simulink model "KillerWhaleModel"  (R2020b)
settings: Solver=ode15s  StartTime=0.0  StopTime=10.0  MaxStep=0.01  RelTol=1e-3
model workspace: external: MATLAB File KillerWhaleParams.m (data not in the file)
undefined symbols (not defined in the file or in its folder): frontParams, rearParams, standParams, X, Y, Z
libraries: sm_lib x4076, nesl_utility x6
(part 2 of 62)

== system KillerWhaleModel/WhaleStand ==
  J5 : Inport
  PitchLink1_1 : Subsystem
      settings: PortSchema="{\"entries\":[{\"content\":{\"sides\":[{\"content\":{\"connectorIds\":[\"LConn1\"]},\"type\":\"ConnectorPlacement.EquallySpacedRectSide\",\"uuid\":\"daed8036-1c83-499a-be75-c3d6daf1be0e\"},{\"content\":{\"connectorIds\":[\"RConn1\"],\"side\":\"RIGHT\"},\"type\":\"ConnectorPlacement.EquallySpacedRectSide\",\"uuid\":\"d51b8bb5-d322-4cdc-bb54-b3adc448b83e\"},{\"content\":{\"connectorIds\":[],\"side\":\"TOP\"},\"type\":\"ConnectorPlacement.EquallySpacedRectSide\",\"uuid\":\"6033db49-1de1-4080-b1d2-f43e71cbe144\"},{\"content\":{\"connectorIds\":[\"RConn2\",\"RConn3\"],\"side\":\"BOTTOM\"},\"type\":\"ConnectorPlacement.EquallySpacedRectSide\",\"uuid\":\"5e0a4000-b8ff-4240-85b3-c85b6cef6958\"},{\"content\":{\"connectorIds\":[],\"side\":\"HIDDEN\"},\"type\":\"ConnectorPlacement.EquallySpacedRectSide\",\"uuid\":\"849e2ead-7697-44fd-a88a-81f8afad95b9\"}]},\"type\":\"ConnectorPlacement.EquallySpacedConnector\",\"uuid\":\"26ddce31-1319-410d-869c-816121a0afb6\"}],\"packageUris\":[\"http://schema.mathworks.com/mf0/Connector/R2020b\"],\"version\":\"1.0\"}"
  PitchLink2_1 : Subsystem
  PitchLink3_1 : Subsystem
      settings: PortSchema="{\"entries\":[{\"content\":{\"sides\":[{\"content\":{\"connectorIds\":[\"LConn1\"]},\"type\":\"ConnectorPlacement.EquallySpacedRectSide\",\"uuid\":\"ffe909db-c886-4e63-ba46-0b3ec8f48d0a\"},{\"content\":{\"connectorIds\":[\"RConn1\"],\"side\":\"RIGHT\"},\"type\":\"ConnectorPlacement.EquallySpacedRectSide\",\"uuid\":\"77d7e64e-07ff-4cea-8643-07133e8c2799\"},{\"content\":{\"connectorIds\":[\"LConn2\"],\"side\":\"TOP\"},\"type\":\"ConnectorPlacement.EquallySpacedRectSide\",\"uuid\":\"189798a8-90a9-455e-91d8-3d815b26c78b\"},{\"content\":{\"connectorIds\":[\"RConn2\"],\"side\":\"BOTTOM\"},\"type\":\"ConnectorPlacement.EquallySpacedRectSide\",\"uuid\":\"6ca3684c-b3f7-48ad-a60e-7715eeec248c\"},{\"content\":{\"connectorIds\":[],\"side\":\"HIDDEN\"},\"type\":\"ConnectorPlacement.EquallySpacedRectSide\",\"uuid\":\"9488b140-3c37-4540-8da6-f5b0cd01be8e\"}]},\"type\":\"ConnectorPlacement.EquallySpacedConnector\",\"uuid\":\"c943227e-23c5-4cc6-8f81-35f98998dc73\"}],\"packageUris\":[\"http://schema.mathworks.com/mf0/Connector/R2020b\"],\"version\":\"1.0\"}"
  PitchLink4_1 : Subsystem
  Revolute1 : sm_lib/Joints/Revolute Joint  JointMode=Normal  SenseConstraintForce=off  SenseConstraintForceX=off  SenseConstraintForceY=off  SenseConstraintForceZ=off  SenseConstraintTorque=off  SenseConstraintTorqueX=off  SenseConstraintTorqueY=off  SenseConstraintTorqueZ=off  SenseTotalForce=off  SenseTotalForceX=off  SenseTotalForceY=off  SenseTotalForceZ=off  SenseTotalTorque=off  SenseTotalTorqueX=off  SenseTotalTorqueY=off  SenseTotalTorqueZ=off  CompositeWrenchDir=FollowerOnBase  CompositeWrenchFrame=BaseFrame  EquilibriumPosition=0  EquilibriumPositionUnits=deg  SpringStiffness=0  SpringStiffnessUnits=N*m/deg  DampingCoefficient=0  DampingCoefficientUnits=N*m/(deg/s)  TorqueActuationMode=NoTorque  MotionActuationMode=ComputedMotion  SensePosition=off  SenseVelocity=off  SenseAcceleration=off  SenseTorqueForce=off  SenseLowerLimitTorqueForce=off  SenseUpperLimitTorqueForce=off  LowerLimitSpecify=off  LowerLimitBound=-90  LowerLimitBoundUnits=deg  LowerLimitStiffness=1e4  LowerLimitStiffnessUnits=N*m/deg  LowerLimitDamping=10  LowerLimitDampingUnits=N*m/(deg/s)  LowerLimitTransitionRegionWidth=0.1  LowerLimitTransitionRegionWidthUnits=deg  UpperLimitSpecify=off  UpperLimitBound=90  UpperLimitBoundUnits=deg  UpperLimitStiffness=1e4  UpperLimitStiffnessUnits=N*m/deg  UpperLimitDamping=10  UpperLimitDampingUnits=N*m/(deg/s)  UpperLimitTransitionRegionWidth=0.1  UpperLimitTransitionRegionWidthUnits=deg  PositionTargetSpecify=off  PositionTargetPriority=Low  PositionTargetValue=standParams.RevoluteJoint(1).Rz.Pos  PositionTargetValueUnits=deg  VelocityTargetSpecify=off  VelocityTargetPriority=High  VelocityTargetValue=0  VelocityTargetValueUnits=deg/s
  Revolute2 : sm_lib/Joints/Revolute Joint  JointMode=Normal  SenseConstraintForce=off  SenseConstraintForceX=off  SenseConstraintForceY=off  SenseConstraintForceZ=off  SenseConstraintTorque=off  SenseConstraintTorqueX=off  SenseConstraintTorqueY=off  SenseConstraintTorqueZ=off  SenseTotalForce=off  SenseTotalForceX=off  SenseTotalForceY=off  SenseTotalForceZ=off  SenseTotalTorque=off  SenseTotalTorqueX=off  SenseTotalTorqueY=off  SenseTotalTorqueZ=off  CompositeWrenchDir=FollowerOnBase  CompositeWrenchFrame=BaseFrame  EquilibriumPosition=0  EquilibriumPositionUnits=deg  SpringStiffness=0  SpringStiffnessUnits=N*m/deg  DampingCoefficient=0  DampingCoefficientUnits=N*m/(deg/s)  TorqueActuationMode=NoTorque  MotionActuationMode=ComputedMotion  SensePosition=off  SenseVelocity=off  SenseAcceleration=off  SenseTorqueForce=off  SenseLowerLimitTorqueForce=off  SenseUpperLimitTorqueForce=off  LowerLimitSpecify=off  LowerLimitBound=-90  LowerLimitBoundUnits=deg  LowerLimitStiffness=1e4  LowerLimitStiffnessUnits=N*m/deg  LowerLimitDamping=10  LowerLimitDampingUnits=N*m/(deg/s)  LowerLimitTransitionRegionWidth=0.1  LowerLimitTransitionRegionWidthUnits=deg  UpperLimitSpecify=off  UpperLimitBound=90  UpperLimitBoundUnits=deg  UpperLimitStiffness=1e4  UpperLimitStiffnessUnits=N*m/deg  UpperLimitDamping=10  UpperLimitDampingUnits=N*m/(deg/s)  UpperLimitTransitionRegionWidth=0.1  UpperLimitTransitionRegionWidthUnits=deg  PositionTargetSpecify=off  PositionTargetPriority=High  PositionTargetValue=0  PositionTargetValueUnits=deg  VelocityTargetSpecify=off  VelocityTargetPriority=High  VelocityTargetValue=0  VelocityTargetValueUnits=deg/s
  Revolute3 : sm_lib/Joints/Revolute Joint  JointMode=Normal  SenseConstraintForce=off  SenseConstraintForceX=off  SenseConstraintForceY=off  SenseConstraintForceZ=off  SenseConstraintTorque=off  SenseConstraintTorqueX=off  SenseConstraintTorqueY=off  SenseConstraintTorqueZ=off  SenseTotalForce=off  SenseTotalForceX=off  SenseTotalForceY=off  SenseTotalForceZ=off  SenseTotalTorque=off  SenseTotalTorqueX=off  SenseTotalTorqueY=off  SenseTotalTorqueZ=off  CompositeWrenchDir=FollowerOnBase  CompositeWrenchFrame=BaseFrame  EquilibriumPosition=0  EquilibriumPositionUnits=deg  SpringStiffness=0  SpringStiffnessUnits=N*m/deg  DampingCoefficient=0  DampingCoefficientUnits=N*m/(deg/s)  TorqueActuationMode=NoTorque  MotionActuationMode=ComputedMotion  SensePosition=off  SenseVelocity=off  SenseAcceleration=off  SenseTorqueForce=off  SenseLowerLimitTorqueForce=off  SenseUpperLimitTorqueForce=off  LowerLimitSpecify=off  LowerLimitBound=-90  LowerLimitBoundUnits=deg  LowerLimitStiffness=1e4  LowerLimitStiffnessUnits=N*m/deg  LowerLimitDamping=10  LowerLimitDampingUnits=N*m/(deg/s)  LowerLimitTransitionRegionWidth=0.1  LowerLimitTransitionRegionWidthUnits=deg  UpperLimitSpecify=off  UpperLimitBound=90  UpperLimitBoundUnits=deg  UpperLimitStiffness=1e4  UpperLimitStiffnessUnits=N*m/deg  UpperLimitDamping=10  UpperLimitDampingUnits=N*m/(deg/s)  UpperLimitTransitionRegionWidth=0.1  UpperLimitTransitionRegionWidthUnits=deg  PositionTargetSpecify=on  PositionTargetPriority=Low  PositionTargetValue=standParams.RevoluteJoint(3).Rz.Pos  PositionTargetValueUnits=deg  VelocityTargetSpecify=off  VelocityTargetPriority=High  VelocityTargetValue=0  VelocityTargetValueUnits=deg/s
  Revolute4 : sm_lib/Joints/Revolute Joint  JointMode=Normal  SenseConstraintForce=off  SenseConstraintForceX=off  SenseConstraintForceY=off  SenseConstraintForceZ=off  SenseConstraintTorque=off  SenseConstraintTorqueX=off  SenseConstraintTorqueY=off  SenseConstraintTorqueZ=off  SenseTotalForce=off  SenseTotalForceX=off  SenseTotalForceY=off  SenseTotalForceZ=off  SenseTotalTorque=off  SenseTotalTorqueX=off  SenseTotalTorqueY=off  SenseTotalTorqueZ=off  CompositeWrenchDir=FollowerOnBase  CompositeWrenchFrame=BaseFrame  EquilibriumPosition=0  EquilibriumPositionUnits=deg  SpringStiffness=0  SpringStiffnessUnits=N*m/deg  DampingCoefficient=0  DampingCoefficientUnits=N*m/(deg/s)  TorqueActuationMode=ComputedTorque  MotionActuationMode=InputMotion  SensePosition=off  SenseVelocity=off  SenseAcceleration=off  SenseTorqueForce=off  SenseLowerLimitTorqueForce=off  SenseUpperLimitTorqueForce=off  LowerLimitSpecify=on  LowerLimitBound=-12.5  LowerLimitBoundUnits=deg  LowerLimitStiffness=1e4  LowerLimitStiffnessUnits=N*m/deg  LowerLimitDamping=1e3  LowerLimitDampingUnits=N*m/(deg/s)  LowerLimitTransitionRegionWidth=0.5  LowerLimitTransitionRegionWidthUnits=deg  UpperLimitSpecify=on  UpperLimitBound=41.5  UpperLimitBoundUnits=deg  UpperLimitStiffness=1e4  UpperLimitStiffnessUnits=N*m/deg  UpperLimitDamping=1e3  UpperLimitDampingUnits=N*m/(deg/s)  UpperLimitTransitionRegionWidth=0.5  UpperLimitTransitionRegionWidthUnits=deg  PositionTargetSpecify=on  PositionTargetPriority=Low  PositionTargetValue=standParams.RevoluteJoint(2).Rz.Pos  PositionTargetValueUnits=deg  VelocityTargetSpecify=off  VelocityTargetPriority=High  VelocityTargetValue=0  VelocityTargetValueUnits=deg/s
  Simulink-PS Converter : nesl_utility/Simulink-PS Converter  PhysicalDomain=network_engine_domain  SubClassName=ps_input  LeftPortType=input  RightPortType=output  PseudoPeriodic=off  Frequencies=[]  NoiseDistribution=none  NoiseParameters=[]  Unit=deg  AffineConversion=off  FilteringAndDerivatives=filter  SimscapeFilterOrder=2  InputFilterTimeConstant=0.01  UdotUserProvided=0
  S1 : PMIOPort  Side=Left
  S2 : PMIOPort  Port=2  Side=Left
  wires:
  J5/1 -> Simulink-PS Converter/1
  connections:
  PitchLink3_1/LConn1 -- Revolute3/RConn1
  PitchLink1_1/LConn1 -- Revolute2/RConn1
  PitchLink2_1/RConn2 -- Revolute3/LConn1
  PitchLink4_1/LConn1 -- Revolute4/RConn1
  PitchLink2_1/RConn1 -- Revolute2/LConn1
  PitchLink4_1/LConn2 -- Revolute1/RConn1
  PitchLink1_1/RConn1 -- Revolute4/LConn1
  PitchLink3_1/RConn1 -- Revolute1/LConn1
  S1/RConn1 -- PitchLink3_1/RConn2
  PitchLink4_1/RConn1 -- S2/RConn1
  Simulink-PS Converter/RConn1 -- Revolute4/LConn2

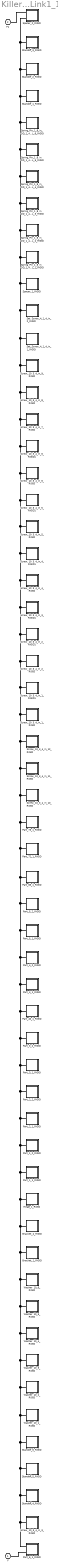
== system KillerWhaleModel/HeadLinkage/HeadLink1_1 ==
  Bracket_1_RIGID : Subsystem
  Bracket_2_RIGID : Subsystem
  Hinge_1_RIGID : Subsystem
  Part_1_1_RIGID : Subsystem
  Part_1_2_RIGID : Subsystem
  Part_2_1_RIGID : Subsystem
  Part_2_2_RIGID : Subsystem
  Part_3_1_RIGID : Subsystem
  Part_3_2_RIGID : Subsystem
  Part_40_1_RIGID : Subsystem
  Part_4_1_RIGID : Subsystem
  Part_4_2_RIGID : Subsystem
  Part_5_1_RIGID : Subsystem
  Part_5_2_RIGID : Subsystem
  Part_65_1_RIGID : Subsystem
  Part_6_1_RIGID : Subsystem
  Part_72_1_RIGID : Subsystem
  Part_73_1_RIGID : Subsystem
  Screw_10_3_4_in_10_RIGID : Subsystem
  Screw_10_3_4_in_11_RIGID : Subsystem
  Screw_10_3_4_in_12_RIGID : Subsystem
  Screw_10_3_4_in_1_RIGID : Subsystem
  Screw_10_3_4_in_1_RIGID1 : Subsystem
  Screw_10_3_4_in_2_RIGID : Subsystem
  Screw_10_3_4_in_2_RIGID1 : Subsystem
  Screw_10_3_4_in_3_RIGID : Subsystem
  Screw_10_3_4_in_3_RIGID1 : Subsystem
  Screw_10_3_4_in_4_RIGID : Subsystem
  Screw_10_3_4_in_4_RIGID1 : Subsystem
  Screw_10_3_4_in_5_RIGID : Subsystem
  Screw_10_3_4_in_5_RIGID1 : Subsystem
  Screw_10_3_4_in_6_RIGID : Subsystem
  Screw_10_3_4_in_6_RIGID1 : Subsystem
  Screw_10_3_4_in_7_RIGID : Subsystem
  Screw_10_3_4_in_8_RIGID : Subsystem
  Screw_10_3_4_in_9_RIGID : Subsystem
  Set_Screw_4_1_4_in_1_RIGID : Subsystem
  Set_Screw_4_1_4_in_2_RIGID : Subsystem
  Spacer_1_RIGID : Subsystem
  Spacer_2_RIGID : Subsystem
  Spring_Pin_1_8_in_OD_1_4_in_L_1_RIGID : Subsystem
  Spring_Pin_1_8_in_OD_1_4_in_L_2_RIGID : Subsystem
  Spring_Pin_1_8_in_OD_1_4_in_L_3_RIGID : Subsystem
  Spring_Pin_1_8_in_OD_1_4_in_L_4_RIGID : Subsystem
  Spring_Pin_1_8_in_OD_1_4_in_L_5_RIGID : Subsystem
  Spring_Pin_1_8_in_OD_1_4_in_L_6_RIGID : Subsystem
  Standoff_1_RIGID : Subsystem
  Standoff_2_RIGID : Subsystem
  Standoff_3_RIGID : Subsystem
  Standoff_4_RIGID : Subsystem
  Standoff_5_RIGID : Subsystem
  Standoff_6_RIGID : Subsystem
  Washer_10_1_RIGID : Subsystem
  Washer_10_2_RIGID : Subsystem
  Washer_10_3_RIGID : Subsystem
  Washer_10_4_RIGID : Subsystem
  Washer_10_5_RIGID : Subsystem
  Washer_10_6_RIGID : Subsystem
  F : PMIOPort  Side=Left
  F1 : PMIOPort  Port=2  Side=Right
  connections:
  Bracket_1_RIGID/LConn1 -- Part_6_1_RIGID/LConn1 -- Screw_10_3_4_in_3_RIGID/LConn1 -- Standoff_4_RIGID/LConn1 -- Standoff_5_RIGID/LConn1 -- Standoff_6_RIGID/LConn1 -- Washer_10_1_RIGID/LConn1 -- Washer_10_2_RIGID/LConn1 -- Washer_10_3_RIGID/LConn1 -- Washer_10_4_RIGID/LConn1 -- Washer_10_5_RIGID/LConn1 -- Washer_10_6_RIGID/LConn1 -- Spacer_2_RIGID/LConn2 -- Standoff_3_RIGID/LConn1 -- Standoff_2_RIGID/LConn1 -- Standoff_1_RIGID/LConn1 -- Spring_Pin_1_8_in_OD_1_4_in_L_6_RIGID/LConn1 -- Spring_Pin_1_8_in_OD_1_4_in_L_5_RIGID/LConn1 -- Spring_Pin_1_8_in_OD_1_4_in_L_4_RIGID/LConn1 -- Spring_Pin_1_8_in_OD_1_4_in_L_3_RIGID/LConn1 -- Spring_Pin_1_8_in_OD_1_4_in_L_2_RIGID/LConn1 -- Spring_Pin_1_8_in_OD_1_4_in_L_1_RIGID/LConn1 -- Spacer_1_RIGID/LConn1 -- Set_Screw_4_1_4_in_2_RIGID/LConn1 -- Set_Screw_4_1_4_in_1_RIGID/LConn1 -- Screw_10_3_4_in_9_RIGID/LConn1 -- Screw_10_3_4_in_8_RIGID/LConn1 -- Screw_10_3_4_in_7_RIGID/LConn1 -- Screw_10_3_4_in_6_RIGID1/LConn1 -- Screw_10_3_4_in_6_RIGID/LConn1 -- Screw_10_3_4_in_5_RIGID1/LConn1 -- Screw_10_3_4_in_5_RIGID/LConn1 -- Screw_10_3_4_in_4_RIGID1/LConn1 -- Screw_10_3_4_in_4_RIGID/LConn1 -- Screw_10_3_4_in_3_RIGID1/LConn1 -- Screw_10_3_4_in_2_RIGID1/LConn1 -- Screw_10_3_4_in_2_RIGID/LConn1 -- Screw_10_3_4_in_1_RIGID1/LConn1 -- Screw_10_3_4_in_1_RIGID/LConn1 -- Screw_10_3_4_in_12_RIGID/LConn1 -- Screw_10_3_4_in_11_RIGID/LConn1 -- Screw_10_3_4_in_10_RIGID/LConn1 -- Part_73_1_RIGID/LConn1 -- Part_72_1_RIGID/LConn1 -- Part_65_1_RIGID/LConn1 -- Part_5_2_RIGID/LConn1 -- Part_5_1_RIGID/LConn1 -- Part_4_2_RIGID/LConn1 -- Part_4_1_RIGID/LConn1 -- Part_40_1_RIGID/LConn1 -- Part_3_2_RIGID/LConn1 -- Part_3_1_RIGID/LConn1 -- Part_2_2_RIGID/LConn1 -- Part_2_1_RIGID/LConn1 -- Part_1_2_RIGID/LConn1 -- Part_1_1_RIGID/LConn1 -- Hinge_1_RIGID/LConn1 -- Bracket_2_RIGID/LConn1
  Part_6_1_RIGID/LConn2 -- F/RConn1
  Spacer_2_RIGID/LConn1 -- F1/RConn1

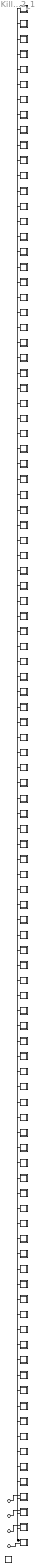
== system KillerWhaleModel/HeadLinkage/HeadLink2_1 ==
  Frame_Part_1_RIGID : Subsystem
  Frame_Part_2_RIGID : Subsystem
  Part_1_1_RIGID : Subsystem
  Part_1_2_RIGID : Subsystem
  Part_1_3_RIGID : Subsystem
  Part_1_4_RIGID : Subsystem
  Part_24_1_RIGID : Subsystem
  Part_24r_1_RIGID : Subsystem
  Part_2_1_RIGID : Subsystem
  Part_2_2_RIGID : Subsystem
  Part_2_3_RIGID : Subsystem
  Part_2_4_RIGID : Subsystem
  Part_3_1_RIGID : Subsystem
  Part_3_2_RIGID : Subsystem
  Part_3_3_RIGID : Subsystem
  Part_3_4_RIGID : Subsystem
  Part_4_1_RIGID : Subsystem
  Part_4_2_RIGID : Subsystem
  Part_4_3_RIGID : Subsystem
  Part_4_4_RIGID : Subsystem
  Part_5_1_RIGID : Subsystem
  Part_5_2_RIGID : Subsystem
  Part_5_3_RIGID : Subsystem
  Part_5_4_RIGID : Subsystem
  Part_6_1_RIGID : Subsystem
  Part_6_2_RIGID : Subsystem
  Part_809_1_RIGID : Subsystem
  Part_809_2_RIGID : Subsystem
  Part_809_3_RIGID : Subsystem
  Part_809_4_RIGID : Subsystem
  Part_809_5_RIGID : Subsystem
  Part_811_1_RIGID : Subsystem
  Part_812_1_RIGID : Subsystem
  Part_813_1_RIGID : Subsystem
  Part_814_1_RIGID : Subsystem
  Part_815_1_RIGID : Subsystem
  Part_816_1_RIGID : Subsystem
  Part_817_1_RIGID : Subsystem
  Part_818_1_RIGID : Subsystem
  Part_819_1_RIGID : Subsystem
  Part_820_1_RIGID : Subsystem
  Part_821_1_RIGID : Subsystem
  Part_822_1_RIGID : Subsystem
  Part_823_1_RIGID : Subsystem
  Part_824_1_RIGID : Subsystem
  Part_824_2_RIGID : Subsystem
  Part_825_1_RIGID : Subsystem
  Part_825_2_RIGID : Subsystem
  Part_826_1_RIGID : Subsystem
  Part_826_2_RIGID : Subsystem
  Part_827_1_RIGID : Subsystem
  Part_827_2_RIGID : Subsystem
  Part_828_1_RIGID : Subsystem
  Part_828_2_RIGID : Subsystem
  Part_867_1_RIGID : Subsystem
  Part_870_1_RIGID : Subsystem
  Part_875_1_RIGID : Subsystem
  Part_936_1_RIGID : Subsystem
  Part_937_1_RIGID : Subsystem
  Part_938_1_RIGID : Subsystem
  Part_939_1_RIGID : Subsystem
  ReferenceFrame : sm_lib/Frames and Transforms/Reference Frame
  Screw_10_3_4_in_1_RIGID : Subsystem
  Screw_10_3_4_in_2_RIGID : Subsystem
  Screw_10_3_4_in_3_RIGID : Subsystem
  Screw_10_3_4_in_4_RIGID : Subsystem
  Screw_10_3_4_in_5_RIGID : Subsystem
  Screw_10_3_4_in_6_RIGID : Subsystem
  Screw_8_1_2_in_1_RIGID : Subsystem
  Screw_8_1_2_in_2_RIGID : Subsystem
  Spring_Pin_1_8_in_OD_1_4_in_L_1_RIGID : Subsystem
  Spring_Pin_1_8_in_OD_1_4_in_L_2_RIGID : Subsystem
  Spring_Pin_1_8_in_OD_1_4_in_L_3_RIGID : Subsystem
  Spring_Pin_1_8_in_OD_1_4_in_L_4_RIGID : Subsystem
  Spring_Pin_1_8_in_OD_1_4_in_L_5_RIGID : Subsystem
  Spring_Pin_1_8_in_OD_1_4_in_L_6_RIGID : Subsystem
  Standoff_1_RIGID : Subsystem
  Washer_10_10_RIGID : Subsystem
  Washer_10_1_RIGID : Subsystem
  Washer_10_2_RIGID : Subsystem
  Washer_10_3_RIGID : Subsystem
  Washer_10_4_RIGID : Subsystem
  Washer_10_5_RIGID : Subsystem
  Washer_10_6_RIGID : Subsystem
  Washer_10_7_RIGID : Subsystem
  Washer_10_8_RIGID : Subsystem
  Washer_10_9_RIGID : Subsystem
  Washer_8_1_RIGID : Subsystem
  Washer_8_2_RIGID : Subsystem
  bulkheads7_1_RIGID : Subsystem
  bulkheads7_2_RIGID : Subsystem
  bulkheads7_3_RIGID : Subsystem
  bulkheads7_4_RIGID : Subsystem
  bulkheads7_5_RIGID : Subsystem
  bulkheads8_1_RIGID : Subsystem
  bulkheads8_2_RIGID : Subsystem
  bulkheads8_3_RIGID : Subsystem
  bulkheads8_4_RIGID : Subsystem
  bulkheads8_5_RIGID : Subsystem
  nut_1_RIGID : Subsystem
  nut_2_RIGID : Subsystem
  nut_3_RIGID : Subsystem
  nut_4_RIGID : Subsystem
  F2 : PMIOPort  Side=Left
  F1 : PMIOPort  Port=2  Side=Left
  F4 : PMIOPort  Port=3  Side=Right
  F : PMIOPort  Port=4  Side=Right
  connections:
  Frame_Part_1_RIGID/LConn1 -- Frame_Part_2_RIGID/LConn2 -- Part_1_1_RIGID/LConn1 -- Part_1_2_RIGID/LConn1 -- Part_1_3_RIGID/LConn2 -- Part_1_4_RIGID/LConn2 -- Part_24_1_RIGID/LConn1 -- Part_24r_1_RIGID/LConn1 -- Part_2_1_RIGID/LConn1 -- Part_2_2_RIGID/LConn1 -- Part_2_3_RIGID/LConn1 -- Part_2_4_RIGID/LConn1 -- Part_3_1_RIGID/LConn1 -- Part_3_2_RIGID/LConn1 -- Part_3_3_RIGID/LConn1 -- Part_3_4_RIGID/LConn1 -- Part_4_1_RIGID/LConn1 -- Part_4_2_RIGID/LConn1 -- Part_4_3_RIGID/LConn1 -- Part_4_4_RIGID/LConn1 -- Part_5_1_RIGID/LConn1 -- Part_5_2_RIGID/LConn1 -- Part_5_3_RIGID/LConn1 -- Part_5_4_RIGID/LConn1 -- Part_6_1_RIGID/LConn1 -- Part_6_2_RIGID/LConn1 -- Part_809_1_RIGID/LConn1 -- Part_809_2_RIGID/LConn1 -- Part_809_3_RIGID/LConn1 -- Part_809_4_RIGID/LConn1 -- Part_809_5_RIGID/LConn1 -- Part_811_1_RIGID/LConn1 -- Part_812_1_RIGID/LConn1 -- Part_813_1_RIGID/LConn1 -- Part_814_1_RIGID/LConn1 -- Part_815_1_RIGID/LConn1 -- Part_816_1_RIGID/LConn1 -- Part_817_1_RIGID/LConn1 -- Part_818_1_RIGID/LConn1 -- Part_819_1_RIGID/LConn1 -- Part_820_1_RIGID/LConn1 -- Part_821_1_RIGID/LConn1 -- Part_822_1_RIGID/LConn1 -- Part_823_1_RIGID/LConn1 -- Part_824_1_RIGID/LConn1 -- Part_824_2_RIGID/LConn1 -- Part_825_1_RIGID/LConn1 -- Part_825_2_RIGID/LConn1 -- Part_826_1_RIGID/LConn1 -- Part_826_2_RIGID/LConn1 -- Part_827_1_RIGID/LConn1 -- Part_827_2_RIGID/LConn1 -- Part_828_1_RIGID/LConn1 -- Part_828_2_RIGID/LConn1 -- Part_867_1_RIGID/LConn1 -- Part_870_1_RIGID/LConn1 -- Part_875_1_RIGID/LConn1 -- Part_936_1_RIGID/LConn1 -- Part_937_1_RIGID/LConn1 -- Part_938_1_RIGID/LConn1 -- Part_939_1_RIGID/LConn1 -- Screw_10_3_4_in_1_RIGID/LConn1 -- Screw_10_3_4_in_2_RIGID/LConn1 -- Screw_10_3_4_in_3_RIGID/LConn1 -- Screw_10_3_4_in_4_RIGID/LConn1 -- Screw_10_3_4_in_5_RIGID/LConn1 -- Screw_10_3_4_in_6_RIGID/LConn1 -- Screw_8_1_2_in_1_RIGID/LConn1 -- Screw_8_1_2_in_2_RIGID/LConn1 -- Spring_Pin_1_8_in_OD_1_4_in_L_1_RIGID/LConn1 -- Spring_Pin_1_8_in_OD_1_4_in_L_2_RIGID/LConn1 -- Spring_Pin_1_8_in_OD_1_4_in_L_3_RIGID/LConn1 -- Spring_Pin_1_8_in_OD_1_4_in_L_4_RIGID/LConn1 -- Spring_Pin_1_8_in_OD_1_4_in_L_5_RIGID/LConn1 -- Spring_Pin_1_8_in_OD_1_4_in_L_6_RIGID/LConn1 -- Standoff_1_RIGID/LConn1 -- Washer_10_10_RIGID/LConn1 -- Washer_10_1_RIGID/LConn1 -- Washer_10_2_RIGID/LConn1 -- Washer_10_3_RIGID/LConn1 -- Washer_10_4_RIGID/LConn1 -- Washer_10_5_RIGID/LConn1 -- Washer_10_6_RIGID/LConn1 -- Washer_10_7_RIGID/LConn1 -- Washer_10_8_RIGID/LConn1 -- Washer_10_9_RIGID/LConn1 -- Washer_8_1_RIGID/LConn1 -- Washer_8_2_RIGID/LConn1 -- bulkheads7_1_RIGID/LConn1 -- bulkheads7_2_RIGID/LConn1 -- bulkheads7_3_RIGID/LConn1 -- bulkheads7_4_RIGID/LConn1 -- bulkheads7_5_RIGID/LConn1 -- bulkheads8_1_RIGID/LConn1 -- bulkheads8_2_RIGID/LConn1 -- bulkheads8_3_RIGID/LConn1 -- bulkheads8_4_RIGID/LConn1 -- bulkheads8_5_RIGID/LConn1 -- nut_1_RIGID/LConn1 -- nut_2_RIGID/LConn1 -- nut_3_RIGID/LConn1 -- nut_4_RIGID/LConn1
  Part_1_4_RIGID/LConn1 -- F/RConn1
  Frame_Part_1_RIGID/LConn2 -- F1/RConn1
  Frame_Part_2_RIGID/LConn1 -- F2/RConn1
  Part_1_3_RIGID/LConn1 -- F4/RConn1

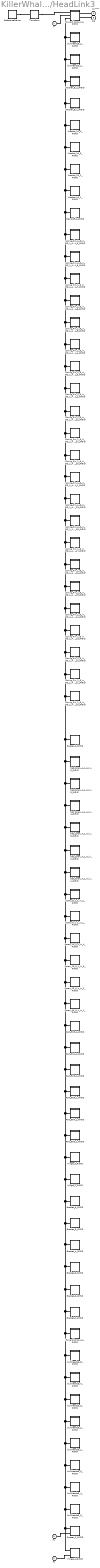
== system KillerWhaleModel/HeadLinkage/HeadLink3_1 ==
  Bracket_1_RIGID : Subsystem
  Bracket_2_RIGID : Subsystem
  Bracket_3_RIGID : Subsystem
  Bracket_4_RIGID : Subsystem
  Bracket_5_RIGID : Subsystem
  Bracket_6_RIGID : Subsystem
  Hinge_1_RIGID : Subsystem
  Hinge_2_RIGID : Subsystem
  Hinge_3_RIGID : Subsystem
  Part_853_1_RIGID : Subsystem
  Part_854_1_RIGID : Subsystem
  Part_855_1_RIGID : Subsystem
  Part_923_1_RIGID : Subsystem
  Part_924_1_RIGID : Subsystem
  Part_925_1_RIGID : Subsystem
  ReferenceFrame : sm_lib/Frames and Transforms/Reference Frame
  Screw_10_3_4_in_1_RIGID : Subsystem
  Screw_10_3_4_in_2_RIGID : Subsystem
  Screw_10_3_4_in_3_RIGID : Subsystem
  Screw_10_3_4_in_4_RIGID : Subsystem
  Screw_8_1_2_in_1_RIGID : Subsystem
  Screw_8_1_2_in_2_RIGID : Subsystem
  Set_Screw_4_1_4_in_1_RIGID : Subsystem
  Set_Screw_4_1_4_in_2_RIGID : Subsystem
  Set_Screw_4_1_4_in_3_RIGID : Subsystem
  Set_Screw_4_1_4_in_4_RIGID : Subsystem
  Set_Screw_4_1_4_in_5_RIGID : Subsystem
  Set_Screw_4_1_4_in_6_RIGID : Subsystem
  Spacer_1_RIGID : Subsystem
  Spacer_2_RIGID : Subsystem
  Spring_Pin_1_8_in_OD_1_4_in_L_10_RIGID : Subsystem
  Spring_Pin_1_8_in_OD_1_4_in_L_11_RIGID : Subsystem
  Spring_Pin_1_8_in_OD_1_4_in_L_12_RIGID : Subsystem
  Spring_Pin_1_8_in_OD_1_4_in_L_13_RIGID : Subsystem
  Spring_Pin_1_8_in_OD_1_4_in_L_14_RIGID : Subsystem
  Spring_Pin_1_8_in_OD_1_4_in_L_15_RIGID : Subsystem
  Spring_Pin_1_8_in_OD_1_4_in_L_16_RIGID : Subsystem
  Spring_Pin_1_8_in_OD_1_4_in_L_17_RIGID : Subsystem
  Spring_Pin_1_8_in_OD_1_4_in_L_18_RIGID : Subsystem
  Spring_Pin_1_8_in_OD_1_4_in_L_19_RIGID : Subsystem
  Spring_Pin_1_8_in_OD_1_4_in_L_1_RIGID : Subsystem
  Spring_Pin_1_8_in_OD_1_4_in_L_20_RIGID : Subsystem
  Spring_Pin_1_8_in_OD_1_4_in_L_21_RIGID : Subsystem
  Spring_Pin_1_8_in_OD_1_4_in_L_22_RIGID : Subsystem
  Spring_Pin_1_8_in_OD_1_4_in_L_2_RIGID : Subsystem
  Spring_Pin_1_8_in_OD_1_4_in_L_3_RIGID : Subsystem
  Spring_Pin_1_8_in_OD_1_4_in_L_4_RIGID : Subsystem
  Spring_Pin_1_8_in_OD_1_4_in_L_5_RIGID : Subsystem
  Spring_Pin_1_8_in_OD_1_4_in_L_6_RIGID : Subsystem
  Spring_Pin_1_8_in_OD_1_4_in_L_7_RIGID : Subsystem
  Spring_Pin_1_8_in_OD_1_4_in_L_8_RIGID : Subsystem
  Spring_Pin_1_8_in_OD_1_4_in_L_9_RIGID : Subsystem
  Standoff_1_RIGID : Subsystem
  Transform : sm_lib/Frames and Transforms/Rigid Transform  TranslationMethod=Cartesian  TranslationStandardOffset=0  TranslationLengthUnit=in  TranslationStandardAxis=+Z  TranslationCartesianOffset=frontParams.RigidTransform(422).translation  TranslationROffset=0  TranslationROffsetUnits=m  TranslationZOffset=0  TranslationZOffsetUnits=m  TranslationThetaOffset=0  TranslationThetaOffsetUnits=deg  RotationMethod=ArbitraryAxis  RotationAngleUnits=rad  RotationStandardAxis=+Z  RotationAngle=frontParams.RigidTransform(422).angle  RotationArbitraryAxis=frontParams.RigidTransform(422).axis  FollAlignAxisA=+X  BaseAlignAxisA=+Y  FollAlignAxisB=+Y  BaseAlignAxisB=+Z  RotationSequenceAxes=FollowerAxes  RotationSequence=XYX  RotationSequenceAngles=[0 0 0]  RotationSequenceAnglesUnits=deg  RotationMatrix=[1 0 0; 0 1 0; 0 0 1]
  Washer_10_1_RIGID : Subsystem
  Washer_10_2_RIGID : Subsystem
  Washer_10_3_RIGID : Subsystem
  Washer_10_4_RIGID : Subsystem
  Washer_8_1_RIGID : Subsystem
  Washer_8_2_RIGID : Subsystem
  bulkheads5_1_RIGID : Subsystem
  bulkheads5_2_RIGID : Subsystem
  bulkheads5_3_RIGID : Subsystem
  bulkheads5_4_RIGID : Subsystem
  bulkheads5_5_RIGID : Subsystem
  bulkheads6_1_RIGID : Subsystem
  bulkheads6_2_RIGID : Subsystem
  bulkheads6_3_RIGID : Subsystem
  bulkheads6_4_RIGID : Subsystem
  bulkheads6_5_RIGID : Subsystem
  forward_torso_l_1_RIGID : Subsystem
  forward_torso_r_1_RIGID : Subsystem
  F : PMIOPort  Side=Left
  F2 : PMIOPort  Port=2  Side=Left
  F1 : PMIOPort  Port=3  Side=Right
  S2 : PMIOPort  Port=4  Side=Right
  S3 : PMIOPort  Port=5  Side=Right
  connections:
  Bracket_1_RIGID/LConn1 -- Hinge_1_RIGID/LConn1 -- Spacer_2_RIGID/LConn1 -- bulkheads5_3_RIGID/LConn1 -- bulkheads5_4_RIGID/LConn1 -- bulkheads5_5_RIGID/LConn1 -- bulkheads6_1_RIGID/LConn1 -- bulkheads6_2_RIGID/LConn1 -- bulkheads6_3_RIGID/LConn1 -- bulkheads6_4_RIGID/LConn1 -- bulkheads6_5_RIGID/LConn1 -- forward_torso_l_1_RIGID/LConn1 -- bulkheads5_2_RIGID/LConn1 -- forward_torso_r_1_RIGID/LConn3 -- bulkheads5_1_RIGID/LConn1 -- Washer_8_2_RIGID/LConn1 -- Washer_8_1_RIGID/LConn1 -- Washer_10_4_RIGID/LConn1 -- Washer_10_3_RIGID/LConn1 -- Washer_10_2_RIGID/LConn1 -- Washer_10_1_RIGID/LConn1 -- Standoff_1_RIGID/LConn1 -- Spring_Pin_1_8_in_OD_1_4_in_L_9_RIGID/LConn1 -- Spring_Pin_1_8_in_OD_1_4_in_L_8_RIGID/LConn1 -- Spring_Pin_1_8_in_OD_1_4_in_L_7_RIGID/LConn1 -- Spring_Pin_1_8_in_OD_1_4_in_L_6_RIGID/LConn1 -- Spring_Pin_1_8_in_OD_1_4_in_L_5_RIGID/LConn1 -- Spring_Pin_1_8_in_OD_1_4_in_L_4_RIGID/LConn1 -- Spring_Pin_1_8_in_OD_1_4_in_L_3_RIGID/LConn1 -- Spring_Pin_1_8_in_OD_1_4_in_L_2_RIGID/LConn1 -- Spring_Pin_1_8_in_OD_1_4_in_L_22_RIGID/LConn1 -- Spring_Pin_1_8_in_OD_1_4_in_L_21_RIGID/LConn1 -- Spring_Pin_1_8_in_OD_1_4_in_L_20_RIGID/LConn1 -- Spring_Pin_1_8_in_OD_1_4_in_L_1_RIGID/LConn1 -- Spring_Pin_1_8_in_OD_1_4_in_L_19_RIGID/LConn1 -- Spring_Pin_1_8_in_OD_1_4_in_L_18_RIGID/LConn1 -- Spring_Pin_1_8_in_OD_1_4_in_L_17_RIGID/LConn1 -- Spring_Pin_1_8_in_OD_1_4_in_L_16_RIGID/LConn1 -- Spring_Pin_1_8_in_OD_1_4_in_L_15_RIGID/LConn1 -- Spring_Pin_1_8_in_OD_1_4_in_L_14_RIGID/LConn1 -- Spring_Pin_1_8_in_OD_1_4_in_L_13_RIGID/LConn1 -- Spring_Pin_1_8_in_OD_1_4_in_L_12_RIGID/LConn1 -- Spring_Pin_1_8_in_OD_1_4_in_L_11_RIGID/LConn1 -- Spring_Pin_1_8_in_OD_1_4_in_L_10_RIGID/LConn1 -- Spacer_1_RIGID/LConn1 -- Set_Screw_4_1_4_in_6_RIGID/LConn1 -- Set_Screw_4_1_4_in_5_RIGID/LConn1 -- Set_Screw_4_1_4_in_4_RIGID/LConn1 -- Set_Screw_4_1_4_in_3_RIGID/LConn1 -- Set_Screw_4_1_4_in_2_RIGID/LConn1 -- Set_Screw_4_1_4_in_1_RIGID/LConn1 -- Screw_8_1_2_in_2_RIGID/LConn1 -- Screw_8_1_2_in_1_RIGID/LConn1 -- Screw_10_3_4_in_4_RIGID/LConn1 -- Screw_10_3_4_in_3_RIGID/LConn1 -- Screw_10_3_4_in_2_RIGID/LConn1 -- Screw_10_3_4_in_1_RIGID/LConn1 -- Part_925_1_RIGID/LConn1 -- Part_924_1_RIGID/LConn1 -- Part_923_1_RIGID/LConn1 -- Part_855_1_RIGID/LConn1 -- Part_854_1_RIGID/LConn1 -- Part_853_1_RIGID/LConn1 -- Hinge_3_RIGID/LConn1 -- Hinge_2_RIGID/LConn1 -- Bracket_6_RIGID/LConn1 -- Bracket_5_RIGID/LConn1 -- Bracket_4_RIGID/LConn1 -- Bracket_3_RIGID/LConn1 -- Bracket_2_RIGID/LConn1
  forward_torso_r_1_RIGID/LConn2 -- F/RConn1
  Spacer_2_RIGID/LConn2 -- F1/RConn1
  Hinge_1_RIGID/LConn2 -- F2/RConn1
  Transform/RConn1 -- forward_torso_r_1_RIGID/LConn1
  ReferenceFrame/RConn1 -- Transform/LConn1
  S2/RConn1 -- forward_torso_r_1_RIGID/RConn1
  S3/RConn1 -- forward_torso_r_1_RIGID/RConn2

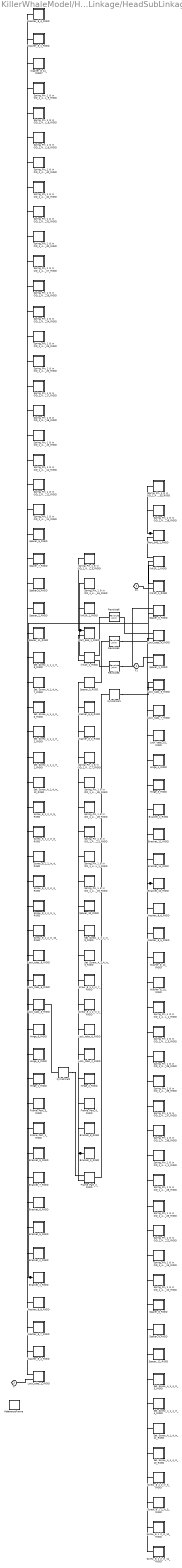
== system KillerWhaleModel/HeadLinkage/HeadSubLinkage_1 ==
  Bracket_10_RIGID : Subsystem
  Bracket_11_RIGID : Subsystem
  Bracket_12_RIGID : Subsystem
  Bracket_1_RIGID : Subsystem
  Bracket_2_RIGID : Subsystem
  Bracket_3_RIGID : Subsystem
  Bracket_4_RIGID : Subsystem
  Bracket_5_RIGID : Subsystem
  Bracket_6_RIGID : Subsystem
  Bracket_7_RIGID : Subsystem
  Bracket_8_RIGID : Subsystem
  Bracket_9_RIGID : Subsystem
  Cylindrical1 : sm_lib/Joints/Cylindrical Joint  JointMode=Normal  SenseConstraintForce=off  SenseConstraintForceX=off  SenseConstraintForceY=off  SenseConstraintForceZ=off  SenseConstraintTorque=off  SenseConstraintTorqueX=off  SenseConstraintTorqueY=off  SenseConstraintTorqueZ=off  SenseTotalForce=off  SenseTotalForceX=off  SenseTotalForceY=off  SenseTotalForceZ=off  SenseTotalTorque=off  SenseTotalTorqueX=off  SenseTotalTorqueY=off  SenseTotalTorqueZ=off  CompositeWrenchDir=FollowerOnBase  CompositeWrenchFrame=BaseFrame  PzEquilibriumPosition=0  PzEquilibriumPositionUnits=m  PzSpringStiffness=0  PzSpringStiffnessUnits=N/m  PzDampingCoefficient=0  PzDampingCoefficientUnits=N/(m/s)  PzTorqueActuationMode=NoTorque  PzMotionActuationMode=ComputedMotion  PzSensePosition=off  PzSenseVelocity=off  PzSenseAcceleration=off  PzSenseTorqueForce=off  PzSenseLowerLimitTorqueForce=off  PzSenseUpperLimitTorqueForce=off  PzLowerLimitSpecify=off  PzLowerLimitBound=-1  PzLowerLimitBoundUnits=m  PzLowerLimitStiffness=1e6  PzLowerLimitStiffnessUnits=N/m  PzLowerLimitDamping=1e3  PzLowerLimitDampingUnits=N/(m/s)  PzLowerLimitTransitionRegionWidth=1e-4  PzLowerLimitTransitionRegionWidthUnits=m  PzUpperLimitSpecify=off  PzUpperLimitBound=1  PzUpperLimitBoundUnits=m  PzUpperLimitStiffness=1e6  PzUpperLimitStiffnessUnits=N/m  PzUpperLimitDamping=1e3  PzUpperLimitDampingUnits=N/(m/s)  PzUpperLimitTransitionRegionWidth=1e-4  PzUpperLimitTransitionRegionWidthUnits=m  PzPositionTargetSpecify=off  PzPositionTargetPriority=High  PzPositionTargetValue=0  PzPositionTargetValueUnits=m  PzVelocityTargetSpecify=off  PzVelocityTargetPriority=High  PzVelocityTargetValue=0  PzVelocityTargetValueUnits=m/s  RzEquilibriumPosition=0  RzEquilibriumPositionUnits=deg  RzSpringStiffness=0  RzSpringStiffnessUnits=N*m/deg  RzDampingCoefficient=0  RzDampingCoefficientUnits=N*m/(deg/s)  RzTorqueActuationMode=NoTorque  RzMotionActuationMode=ComputedMotion  RzSensePosition=off  RzSenseVelocity=off  RzSenseAcceleration=off  RzSenseTorqueForce=off  RzSenseLowerLimitTorqueForce=off  RzSenseUpperLimitTorqueForce=off  RzLowerLimitSpecify=off  RzLowerLimitBound=-90  RzLowerLimitBoundUnits=deg  RzLowerLimitStiffness=1e4  RzLowerLimitStiffnessUnits=N*m/deg  RzLowerLimitDamping=10  RzLowerLimitDampingUnits=N*m/(deg/s)  RzLowerLimitTransitionRegionWidth=0.1  RzLowerLimitTransitionRegionWidthUnits=deg  RzUpperLimitSpecify=off  RzUpperLimitBound=90  RzUpperLimitBoundUnits=deg  RzUpperLimitStiffness=1e4  RzUpperLimitStiffnessUnits=N*m/deg  RzUpperLimitDamping=10  RzUpperLimitDampingUnits=N*m/(deg/s)  RzUpperLimitTransitionRegionWidth=0.1  RzUpperLimitTransitionRegionWidthUnits=deg  RzPositionTargetSpecify=off  RzPositionTargetPriority=High  RzPositionTargetValue=0  RzPositionTargetValueUnits=deg  RzVelocityTargetSpecify=off  RzVelocityTargetPriority=High  RzVelocityTargetValue=0  RzVelocityTargetValueUnits=deg/s
  Cylindrical2 : sm_lib/Joints/Cylindrical Joint  JointMode=Normal  SenseConstraintForce=off  SenseConstraintForceX=off  SenseConstraintForceY=off  SenseConstraintForceZ=off  SenseConstraintTorque=off  SenseConstraintTorqueX=off  SenseConstraintTorqueY=off  SenseConstraintTorqueZ=off  SenseTotalForce=off  SenseTotalForceX=off  SenseTotalForceY=off  SenseTotalForceZ=off  SenseTotalTorque=off  SenseTotalTorqueX=off  SenseTotalTorqueY=off  SenseTotalTorqueZ=off  CompositeWrenchDir=FollowerOnBase  CompositeWrenchFrame=BaseFrame  PzEquilibriumPosition=0  PzEquilibriumPositionUnits=m  PzSpringStiffness=0  PzSpringStiffnessUnits=N/m  PzDampingCoefficient=0  PzDampingCoefficientUnits=N/(m/s)  PzTorqueActuationMode=NoTorque  PzMotionActuationMode=ComputedMotion  PzSensePosition=off  PzSenseVelocity=off  PzSenseAcceleration=off  PzSenseTorqueForce=off  PzSenseLowerLimitTorqueForce=off  PzSenseUpperLimitTorqueForce=off  PzLowerLimitSpecify=off  PzLowerLimitBound=-1  PzLowerLimitBoundUnits=m  PzLowerLimitStiffness=1e6  PzLowerLimitStiffnessUnits=N/m  PzLowerLimitDamping=1e3  PzLowerLimitDampingUnits=N/(m/s)  PzLowerLimitTransitionRegionWidth=1e-4  PzLowerLimitTransitionRegionWidthUnits=m  PzUpperLimitSpecify=off  PzUpperLimitBound=1  PzUpperLimitBoundUnits=m  PzUpperLimitStiffness=1e6  PzUpperLimitStiffnessUnits=N/m  PzUpperLimitDamping=1e3  PzUpperLimitDampingUnits=N/(m/s)  PzUpperLimitTransitionRegionWidth=1e-4  PzUpperLimitTransitionRegionWidthUnits=m  PzPositionTargetSpecify=off  PzPositionTargetPriority=High  PzPositionTargetValue=0  PzPositionTargetValueUnits=m  PzVelocityTargetSpecify=off  PzVelocityTargetPriority=High  PzVelocityTargetValue=0  PzVelocityTargetValueUnits=m/s  RzEquilibriumPosition=0  RzEquilibriumPositionUnits=deg  RzSpringStiffness=0  RzSpringStiffnessUnits=N*m/deg  RzDampingCoefficient=0  RzDampingCoefficientUnits=N*m/(deg/s)  RzTorqueActuationMode=NoTorque  RzMotionActuationMode=ComputedMotion  RzSensePosition=off  RzSenseVelocity=off  RzSenseAcceleration=off  RzSenseTorqueForce=off  RzSenseLowerLimitTorqueForce=off  RzSenseUpperLimitTorqueForce=off  RzLowerLimitSpecify=off  RzLowerLimitBound=-90  RzLowerLimitBoundUnits=deg  RzLowerLimitStiffness=1e4  RzLowerLimitStiffnessUnits=N*m/deg  RzLowerLimitDamping=10  RzLowerLimitDampingUnits=N*m/(deg/s)  RzLowerLimitTransitionRegionWidth=0.1  RzLowerLimitTransitionRegionWidthUnits=deg  RzUpperLimitSpecify=off  RzUpperLimitBound=90  RzUpperLimitBoundUnits=deg  RzUpperLimitStiffness=1e4  RzUpperLimitStiffnessUnits=N*m/deg  RzUpperLimitDamping=10  RzUpperLimitDampingUnits=N*m/(deg/s)  RzUpperLimitTransitionRegionWidth=0.1  RzUpperLimitTransitionRegionWidthUnits=deg  RzPositionTargetSpecify=off  RzPositionTargetPriority=High  RzPositionTargetValue=0  RzPositionTargetValueUnits=deg  RzVelocityTargetSpecify=off  RzVelocityTargetPriority=High  RzVelocityTargetValue=0  RzVelocityTargetValueUnits=deg/s
  Frame_Part_1_RIGID : Subsystem
  Frame_Part_2_RIGID : Subsystem
  Frame_Part_3_RIGID : Subsystem
  Frame_Part_4_RIGID : Subsystem
  Hinge_1_RIGID : Subsystem
  Hinge_2_RIGID : Subsystem
  Hinge_3_RIGID : Subsystem
  Hinge_4_RIGID : Subsystem
  Hinge_5_RIGID : Subsystem
  Hinge_6_RIGID : Subsystem
  Lock_tabs_10_RIGID : Subsystem
  Lock_tabs_1_RIGID : Subsystem
  Lock_tabs_2_RIGID : Subsystem
  Lock_tabs_3_RIGID : Subsystem
  Lock_tabs_4_RIGID : Subsystem
  Lock_tabs_5_RIGID : Subsystem
  Lock_tabs_6_RIGID : Subsystem
  Lock_tabs_7_RIGID : Subsystem
  Lock_tabs_8_RIGID : Subsystem
  Lock_tabs_9_RIGID : Subsystem
  Part_843_1_RIGID : Subsystem
  Part_844_1_RIGID : Subsystem
  ReferenceFrame : sm_lib/Frames and Transforms/Reference Frame
  Revolute3 : sm_lib/Joints/Revolute Joint  JointMode=Normal  SenseConstraintForce=off  SenseConstraintForceX=off  SenseConstraintForceY=off  SenseConstraintForceZ=off  SenseConstraintTorque=off  SenseConstraintTorqueX=off  SenseConstraintTorqueY=off  SenseConstraintTorqueZ=off  SenseTotalForce=off  SenseTotalForceX=off  SenseTotalForceY=off  SenseTotalForceZ=off  SenseTotalTorque=off  SenseTotalTorqueX=off  SenseTotalTorqueY=off  SenseTotalTorqueZ=off  CompositeWrenchDir=FollowerOnBase  CompositeWrenchFrame=BaseFrame  EquilibriumPosition=0  EquilibriumPositionUnits=deg  SpringStiffness=0  SpringStiffnessUnits=N*m/deg  DampingCoefficient=0  DampingCoefficientUnits=N*m/(deg/s)  TorqueActuationMode=NoTorque  MotionActuationMode=ComputedMotion  SensePosition=off  SenseVelocity=off  SenseAcceleration=off  SenseTorqueForce=off  SenseLowerLimitTorqueForce=off  SenseUpperLimitTorqueForce=off  LowerLimitSpecify=off  LowerLimitBound=-90  LowerLimitBoundUnits=deg  LowerLimitStiffness=1e4  LowerLimitStiffnessUnits=N*m/deg  LowerLimitDamping=10  LowerLimitDampingUnits=N*m/(deg/s)  LowerLimitTransitionRegionWidth=0.1  LowerLimitTransitionRegionWidthUnits=deg  UpperLimitSpecify=off  UpperLimitBound=90  UpperLimitBoundUnits=deg  UpperLimitStiffness=1e4  UpperLimitStiffnessUnits=N*m/deg  UpperLimitDamping=10  UpperLimitDampingUnits=N*m/(deg/s)  UpperLimitTransitionRegionWidth=0.1  UpperLimitTransitionRegionWidthUnits=deg  PositionTargetSpecify=on  PositionTargetPriority=Low  PositionTargetValue=frontParams.RevoluteJoint(3).Rz.Pos  PositionTargetValueUnits=deg  VelocityTargetSpecify=off  VelocityTargetPriority=High  VelocityTargetValue=0  VelocityTargetValueUnits=deg/s
  Revolute5 : sm_lib/Joints/Revolute Joint  JointMode=Normal  SenseConstraintForce=off  SenseConstraintForceX=off  SenseConstraintForceY=off  SenseConstraintForceZ=off  SenseConstraintTorque=off  SenseConstraintTorqueX=off  SenseConstraintTorqueY=off  SenseConstraintTorqueZ=off  SenseTotalForce=off  SenseTotalForceX=off  SenseTotalForceY=off  SenseTotalForceZ=off  SenseTotalTorque=off  SenseTotalTorqueX=off  SenseTotalTorqueY=off  SenseTotalTorqueZ=off  CompositeWrenchDir=FollowerOnBase  CompositeWrenchFrame=BaseFrame  EquilibriumPosition=0  EquilibriumPositionUnits=deg  SpringStiffness=0  SpringStiffnessUnits=N*m/deg  DampingCoefficient=0  DampingCoefficientUnits=N*m/(deg/s)  TorqueActuationMode=NoTorque  MotionActuationMode=ComputedMotion  SensePosition=off  SenseVelocity=off  SenseAcceleration=off  SenseTorqueForce=off  SenseLowerLimitTorqueForce=off  SenseUpperLimitTorqueForce=off  LowerLimitSpecify=off  LowerLimitBound=-90  LowerLimitBoundUnits=deg  LowerLimitStiffness=1e4  LowerLimitStiffnessUnits=N*m/deg  LowerLimitDamping=10  LowerLimitDampingUnits=N*m/(deg/s)  LowerLimitTransitionRegionWidth=0.1  LowerLimitTransitionRegionWidthUnits=deg  UpperLimitSpecify=off  UpperLimitBound=90  UpperLimitBoundUnits=deg  UpperLimitStiffness=1e4  UpperLimitStiffnessUnits=N*m/deg  UpperLimitDamping=10  UpperLimitDampingUnits=N*m/(deg/s)  UpperLimitTransitionRegionWidth=0.1  UpperLimitTransitionRegionWidthUnits=deg  PositionTargetSpecify=on  PositionTargetPriority=Low  PositionTargetValue=frontParams.RevoluteJoint(1).Rz.Pos  PositionTargetValueUnits=deg  VelocityTargetSpecify=off  VelocityTargetPriority=High  VelocityTargetValue=0  VelocityTargetValueUnits=deg/s
  Revolute6 : sm_lib/Joints/Revolute Joint  JointMode=Normal  SenseConstraintForce=off  SenseConstraintForceX=off  SenseConstraintForceY=off  SenseConstraintForceZ=off  SenseConstraintTorque=off  SenseConstraintTorqueX=off  SenseConstraintTorqueY=off  SenseConstraintTorqueZ=off  SenseTotalForce=off  SenseTotalForceX=off  SenseTotalForceY=off  SenseTotalForceZ=off  SenseTotalTorque=off  SenseTotalTorqueX=off  SenseTotalTorqueY=off  SenseTotalTorqueZ=off  CompositeWrenchDir=FollowerOnBase  CompositeWrenchFrame=BaseFrame  EquilibriumPosition=0  EquilibriumPositionUnits=deg  SpringStiffness=0  SpringStiffnessUnits=N*m/deg  DampingCoefficient=0  DampingCoefficientUnits=N*m/(deg/s)  TorqueActuationMode=NoTorque  MotionActuationMode=ComputedMotion  SensePosition=off  SenseVelocity=off  SenseAcceleration=off  SenseTorqueForce=off  SenseLowerLimitTorqueForce=off  SenseUpperLimitTorqueForce=off  LowerLimitSpecify=off  LowerLimitBound=-90  LowerLimitBoundUnits=deg  LowerLimitStiffness=1e4  LowerLimitStiffnessUnits=N*m/deg  LowerLimitDamping=10  LowerLimitDampingUnits=N*m/(deg/s)  LowerLimitTransitionRegionWidth=0.1  LowerLimitTransitionRegionWidthUnits=deg  UpperLimitSpecify=off  UpperLimitBound=90  UpperLimitBoundUnits=deg  UpperLimitStiffness=1e4  UpperLimitStiffnessUnits=N*m/deg  UpperLimitDamping=10  UpperLimitDampingUnits=N*m/(deg/s)  UpperLimitTransitionRegionWidth=0.1  UpperLimitTransitionRegionWidthUnits=deg  PositionTargetSpecify=on  PositionTargetPriority=Low  PositionTargetValue=frontParams.RevoluteJoint(2).Rz.Pos  PositionTargetValueUnits=deg  VelocityTargetSpecify=off  VelocityTargetPriority=High  VelocityTargetValue=0  VelocityTargetValueUnits=deg/s
  Screw_8_1_2_in_10_RIGID : Subsystem
  Screw_8_1_2_in_11_RIGID : Subsystem
  Screw_8_1_2_in_12_RIGID : Subsystem
  Screw_8_1_2_in_1_RIGID : Subsystem
  Screw_8_1_2_in_2_RIGID : Subsystem
  Screw_8_1_2_in_3_RIGID : Subsystem
  Screw_8_1_2_in_4_RIGID : Subsystem
  Screw_8_1_2_in_5_RIGID : Subsystem
  Screw_8_1_2_in_6_RIGID : Subsystem
  Screw_8_1_2_in_7_RIGID : Subsystem
  Screw_8_1_2_in_8_RIGID : Subsystem
  Screw_8_1_2_in_9_RIGID : Subsystem
  Set_Screw_4_1_4_in_10_RIGID : Subsystem
  Set_Screw_4_1_4_in_11_RIGID : Subsystem
  Set_Screw_4_1_4_in_12_RIGID : Subsystem
  Set_Screw_4_1_4_in_1_RIGID : Subsystem
  Set_Screw_4_1_4_in_2_RIGID : Subsystem
  Set_Screw_4_1_4_in_3_RIGID : Subsystem
  Set_Screw_4_1_4_in_4_RIGID : Subsystem
  Set_Screw_4_1_4_in_5_RIGID : Subsystem
  Set_Screw_4_1_4_in_6_RIGID : Subsystem
  Set_Screw_4_1_4_in_7_RIGID : Subsystem
  Set_Screw_4_1_4_in_8_RIGID : Subsystem
  Set_Screw_4_1_4_in_9_RIGID : Subsystem
  Spacer_10_RIGID : Subsystem
  Spacer_11_RIGID : Subsystem
  Spacer_12_RIGID : Subsystem
  Spacer_1_RIGID : Subsystem
  Spacer_2_RIGID : Subsystem
  Spacer_3_RIGID : Subsystem
  Spacer_4_RIGID : Subsystem
  Spacer_5_RIGID : Subsystem
  Spacer_6_RIGID : Subsystem
  Spacer_7_RIGID : Subsystem
  Spacer_8_RIGID : Subsystem
  Spacer_9_RIGID : Subsystem
  Spring_Pin_1_8_in_OD_1_4_in_L_10_RIGID : Subsystem
  Spring_Pin_1_8_in_OD_1_4_in_L_11_RIGID : Subsystem
  Spring_Pin_1_8_in_OD_1_4_in_L_12_RIGID : Subsystem
  Spring_Pin_1_8_in_OD_1_4_in_L_13_RIGID : Subsystem
  Spring_Pin_1_8_in_OD_1_4_in_L_14_RIGID : Subsystem
  Spring_Pin_1_8_in_OD_1_4_in_L_15_RIGID : Subsystem
  Spring_Pin_1_8_in_OD_1_4_in_L_16_RIGID : Subsystem
  Spring_Pin_1_8_in_OD_1_4_in_L_17_RIGID : Subsystem
  Spring_Pin_1_8_in_OD_1_4_in_L_18_RIGID : Subsystem
  Spring_Pin_1_8_in_OD_1_4_in_L_19_RIGID : Subsystem
  Spring_Pin_1_8_in_OD_1_4_in_L_1_RIGID : Subsystem
  Spring_Pin_1_8_in_OD_1_4_in_L_20_RIGID : Subsystem
  Spring_Pin_1_8_in_OD_1_4_in_L_21_RIGID : Subsystem
  Spring_Pin_1_8_in_OD_1_4_in_L_22_RIGID : Subsystem
  Spring_Pin_1_8_in_OD_1_4_in_L_23_RIGID : Subsystem
  Spring_Pin_1_8_in_OD_1_4_in_L_24_RIGID : Subsystem
  Spring_Pin_1_8_in_OD_1_4_in_L_25_RIGID : Subsystem
  Spring_Pin_1_8_in_OD_1_4_in_L_26_RIGID : Subsystem
  Spring_Pin_1_8_in_OD_1_4_in_L_27_RIGID : Subsystem
  Spring_Pin_1_8_in_OD_1_4_in_L_28_RIGID : Subsystem
  Spring_Pin_1_8_in_OD_1_4_in_L_29_RIGID : Subsystem
  Spring_Pin_1_8_in_OD_1_4_in_L_2_RIGID : Subsystem
  Spring_Pin_1_8_in_OD_1_4_in_L_30_RIGID : Subsystem
  Spring_Pin_1_8_in_OD_1_4_in_L_31_RIGID : Subsystem
  Spring_Pin_1_8_in_OD_1_4_in_L_32_RIGID : Subsystem
  Spring_Pin_1_8_in_OD_1_4_in_L_33_RIGID : Subsystem
  Spring_Pin_1_8_in_OD_1_4_in_L_34_RIGID : Subsystem
  Spring_Pin_1_8_in_OD_1_4_in_L_35_RIGID : Subsystem
  Spring_Pin_1_8_in_OD_1_4_in_L_36_RIGID : Subsystem
  Spring_Pin_1_8_in_OD_1_4_in_L_37_RIGID : Subsystem
  Spring_Pin_1_8_in_OD_1_4_in_L_38_RIGID : Subsystem
  Spring_Pin_1_8_in_OD_1_4_in_L_39_RIGID : Subsystem
  Spring_Pin_1_8_in_OD_1_4_in_L_3_RIGID : Subsystem
  Spring_Pin_1_8_in_OD_1_4_in_L_40_RIGID : Subsystem
  Spring_Pin_1_8_in_OD_1_4_in_L_4_RIGID : Subsystem
  Spring_Pin_1_8_in_OD_1_4_in_L_5_RIGID : Subsystem
  Spring_Pin_1_8_in_OD_1_4_in_L_6_RIGID : Subsystem
  Spring_Pin_1_8_in_OD_1_4_in_L_7_RIGID : Subsystem
  Spring_Pin_1_8_in_OD_1_4_in_L_8_RIGID : Subsystem
  Spring_Pin_1_8_in_OD_1_4_in_L_9_RIGID : Subsystem
  Washer_8_10_RIGID : Subsystem
  Washer_8_11_RIGID : Subsystem
  Washer_8_12_RIGID : Subsystem
  Washer_8_1_RIGID : Subsystem
  Washer_8_2_RIGID : Subsystem
  Washer_8_3_RIGID : Subsystem
  Washer_8_4_RIGID : Subsystem
  Washer_8_5_RIGID : Subsystem
  Washer_8_6_RIGID : Subsystem
  Washer_8_7_RIGID : Subsystem
  Washer_8_8_RIGID : Subsystem
  Washer_8_9_RIGID : Subsystem
  link1fl_1_RIGID : Subsystem
  link1fr_1_RIGID : Subsystem
  link2fl_1_RIGID : Subsystem
  link2fr_1_RIGID : Subsystem
  F2 : PMIOPort  Side=Left
  F1 : PMIOPort  Port=2  Side=Left
  F : PMIOPort  Port=3  Side=Right
  connections:
  Bracket_1_RIGID/LConn1 -- Bracket_2_RIGID/LConn1 -- Bracket_5_RIGID/LConn1 -- Bracket_6_RIGID/LConn1 -- Bracket_7_RIGID/LConn1 -- Bracket_9_RIGID/LConn1 -- Frame_Part_1_RIGID/LConn1 -- Frame_Part_3_RIGID/LConn1 -- Hinge_1_RIGID/LConn1 -- Hinge_5_RIGID/LConn1 -- Hinge_6_RIGID/LConn1 -- Lock_tabs_1_RIGID/LConn1 -- Lock_tabs_3_RIGID/LConn1 -- Lock_tabs_8_RIGID/LConn1 -- Lock_tabs_9_RIGID/LConn1 -- Screw_8_1_2_in_10_RIGID/LConn1 -- Screw_8_1_2_in_1_RIGID/LConn1 -- Screw_8_1_2_in_3_RIGID/LConn1 -- Screw_8_1_2_in_4_RIGID/LConn1 -- Screw_8_1_2_in_8_RIGID/LConn1 -- Screw_8_1_2_in_9_RIGID/LConn1 -- Set_Screw_4_1_4_in_12_RIGID/LConn1 -- Set_Screw_4_1_4_in_1_RIGID/LConn1 -- Set_Screw_4_1_4_in_2_RIGID/LConn1 -- Set_Screw_4_1_4_in_6_RIGID/LConn1 -- Set_Screw_4_1_4_in_7_RIGID/LConn1 -- Set_Screw_4_1_4_in_8_RIGID/LConn1 -- Spacer_11_RIGID/LConn1 -- Spacer_2_RIGID/LConn1 -- Spacer_5_RIGID/LConn2 -- Spacer_6_RIGID/LConn1 -- Spacer_7_RIGID/LConn1 -- Spacer_9_RIGID/LConn1 -- Spring_Pin_1_8_in_OD_1_4_in_L_11_RIGID/LConn1 -- Spring_Pin_1_8_in_OD_1_4_in_L_12_RIGID/LConn1 -- Spring_Pin_1_8_in_OD_1_4_in_L_14_RIGID/LConn1 -- Spring_Pin_1_8_in_OD_1_4_in_L_15_RIGID/LConn1 -- Spring_Pin_1_8_in_OD_1_4_in_L_16_RIGID/LConn1 -- Spring_Pin_1_8_in_OD_1_4_in_L_17_RIGID/LConn1 -- Spring_Pin_1_8_in_OD_1_4_in_L_20_RIGID/LConn1 -- Spring_Pin_1_8_in_OD_1_4_in_L_23_RIGID/LConn1 -- Spring_Pin_1_8_in_OD_1_4_in_L_24_RIGID/LConn1 -- Spring_Pin_1_8_in_OD_1_4_in_L_26_RIGID/LConn1 -- Spring_Pin_1_8_in_OD_1_4_in_L_27_RIGID/LConn1 -- Spring_Pin_1_8_in_OD_1_4_in_L_30_RIGID/LConn1 -- Spring_Pin_1_8_in_OD_1_4_in_L_31_RIGID/LConn1 -- Spring_Pin_1_8_in_OD_1_4_in_L_32_RIGID/LConn1 -- Spring_Pin_1_8_in_OD_1_4_in_L_40_RIGID/LConn1 -- Spring_Pin_1_8_in_OD_1_4_in_L_6_RIGID/LConn1 -- Spring_Pin_1_8_in_OD_1_4_in_L_8_RIGID/LConn1 -- Spring_Pin_1_8_in_OD_1_4_in_L_9_RIGID/LConn1 -- Washer_8_11_RIGID/LConn1 -- Washer_8_1_RIGID/LConn1 -- Washer_8_3_RIGID/LConn1 -- Washer_8_4_RIGID/LConn1 -- Washer_8_7_RIGID/LConn1 -- Washer_8_9_RIGID/LConn1
  Bracket_10_RIGID/LConn1 -- Bracket_11_RIGID/LConn1 -- Bracket_12_RIGID/LConn1 -- Bracket_4_RIGID/LConn1 -- Hinge_3_RIGID/LConn1 -- Hinge_4_RIGID/LConn1 -- Lock_tabs_10_RIGID/LConn1 -- Lock_tabs_4_RIGID/LConn2 -- Lock_tabs_5_RIGID/LConn2 -- Lock_tabs_7_RIGID/LConn1 -- Screw_8_1_2_in_11_RIGID/LConn1 -- Screw_8_1_2_in_12_RIGID/LConn1 -- Screw_8_1_2_in_5_RIGID/LConn1 -- Screw_8_1_2_in_6_RIGID/LConn1 -- Set_Screw_4_1_4_in_10_RIGID/LConn1 -- Set_Screw_4_1_4_in_11_RIGID/LConn1 -- Set_Screw_4_1_4_in_4_RIGID/LConn1 -- Set_Screw_4_1_4_in_5_RIGID/LConn1 -- Spacer_12_RIGID/LConn1 -- Spacer_1_RIGID/LConn2 -- Spacer_4_RIGID/LConn1 -- Spacer_8_RIGID/LConn1 -- Spring_Pin_1_8_in_OD_1_4_in_L_10_RIGID/LConn1 -- Spring_Pin_1_8_in_OD_1_4_in_L_13_RIGID/LConn1 -- Spring_Pin_1_8_in_OD_1_4_in_L_22_RIGID/LConn1 -- Spring_Pin_1_8_in_OD_1_4_in_L_25_RIGID/LConn1 -- Spring_Pin_1_8_in_OD_1_4_in_L_28_RIGID/LConn1 -- Spring_Pin_1_8_in_OD_1_4_in_L_2_RIGID/LConn1 -- Spring_Pin_1_8_in_OD_1_4_in_L_36_RIGID/LConn1 -- Spring_Pin_1_8_in_OD_1_4_in_L_37_RIGID/LConn1 -- Spring_Pin_1_8_in_OD_1_4_in_L_38_RIGID/LConn1 -- Spring_Pin_1_8_in_OD_1_4_in_L_39_RIGID/LConn1 -- Spring_Pin_1_8_in_OD_1_4_in_L_3_RIGID/LConn1 -- Spring_Pin_1_8_in_OD_1_4_in_L_4_RIGID/LConn1 -- Washer_8_10_RIGID/LConn1 -- Washer_8_12_RIGID/LConn1 -- Washer_8_5_RIGID/LConn1 -- Washer_8_6_RIGID/LConn1
  Revolute5/RConn1 -- Spacer_5_RIGID/LConn1
  Revolute6/LConn1 -- link2fl_1_RIGID/RConn1
  Lock_tabs_4_RIGID/LConn1 -- Revolute6/RConn1
  Cylindrical2/LConn1 -- Lock_tabs_3_RIGID/RConn1
  Cylindrical2/RConn1 -- Frame_Part_2_RIGID/LConn1
  Part_844_1_RIGID/LConn2 -- link2fl_1_RIGID/LConn2
  Revolute3/LConn1 -- Spacer_3_RIGID/RConn1
  Revolute3/RConn1 -- link1fl_1_RIGID/LConn3
  Part_843_1_RIGID/LConn2 -- link1fl_1_RIGID/LConn1
  Lock_tabs_1_RIGID/LConn2 -- F/RConn1
  link1fl_1_RIGID/LConn2 -- link1fr_1_RIGID/LConn1
  Spacer_1_RIGID/LConn1 -- F1/RConn1
  link1fr_1_RIGID/LConn2 -- F2/RConn1
  Part_843_1_RIGID/LConn1 -- Spring_Pin_1_8_in_OD_1_4_in_L_18_RIGID/LConn1 -- Spring_Pin_1_8_in_OD_1_4_in_L_33_RIGID/LConn1
  link2fl_1_RIGID/LConn1 -- link2fr_1_RIGID/LConn1
  Bracket_3_RIGID/LConn1 -- Bracket_8_RIGID/LConn1 -- Frame_Part_2_RIGID/LConn2 -- Frame_Part_4_RIGID/LConn1 -- Hinge_2_RIGID/LConn1 -- Lock_tabs_2_RIGID/LConn1 -- Lock_tabs_6_RIGID/LConn1 -- Screw_8_1_2_in_2_RIGID/LConn1 -- Screw_8_1_2_in_7_RIGID/LConn1 -- Set_Screw_4_1_4_in_3_RIGID/LConn1 -- Set_Screw_4_1_4_in_9_RIGID/LConn1 -- Spacer_10_RIGID/LConn1 -- Spacer_3_RIGID/LConn1 -- Spring_Pin_1_8_in_OD_1_4_in_L_19_RIGID/LConn1 -- Spring_Pin_1_8_in_OD_1_4_in_L_1_RIGID/LConn1 -- Spring_Pin_1_8_in_OD_1_4_in_L_21_RIGID/LConn1 -- Spring_Pin_1_8_in_OD_1_4_in_L_29_RIGID/LConn1 -- Spring_Pin_1_8_in_OD_1_4_in_L_35_RIGID/LConn1 -- Spring_Pin_1_8_in_OD_1_4_in_L_7_RIGID/LConn1 -- Washer_8_2_RIGID/LConn1 -- Washer_8_8_RIGID/LConn1
  Part_844_1_RIGID/LConn1 -- Spring_Pin_1_8_in_OD_1_4_in_L_34_RIGID/LConn1 -- Spring_Pin_1_8_in_OD_1_4_in_L_5_RIGID/LConn1
  Cylindrical1/LConn1 -- Frame_Part_2_RIGID/RConn1
  Cylindrical1/RConn1 -- Lock_tabs_5_RIGID/LConn1
  Revolute5/LConn1 -- link2fl_1_RIGID/RConn2
